simulink model "myTMSI_AnnaSparapani"  (R2017b)
settings: Solver=FixedStepAuto  StartTime=0.0  StopTime=Inf  FixedStep=0.01  RelTol=1e-3
StopFcn:
  | [file,path] = uiputfile;
  | cd(path)
  | save(file, 'EMGdata', 'EMGcount', 'QuatAngle', 'Angles', 'Angles23', 'QuatAngle1')
  | cd ..
libraries: dspindex x8
settings Model: SimulationMode=external  ExtModeTrigDuration=50000  Creator=constantin  LastModifiedBy=root
settings DataIOCC: SaveFormat=Array
settings OptimizationCC: ExpressionDepthLimit=2147483647  LifeSpan=1
settings DebuggingCC: UnderspecifiedInitializationDetection=Classic  MergeDetectMultiDrivingBlocksExec=none  SolverPrmCheckMsg=warning  StateNameClashWarn=warning  SFUnexpectedBacktrackingDiag=warning  SFNoUnconditionalDefaultTransitionDiag=warning  SFExecutionAtInitializationDiag=none
settings HardwareCC: ProdBitPerPointer=32  ProdBitPerSizeT=32  ProdBitPerPtrDiffT=32  ProdLargestAtomicFloat=None  ProdIntDivRoundTo=Undefined  ProdEndianess=Unspecified  ProdWordSize=32  ProdHWDeviceType=32-bit Generic
settings ModelReferenceCC: PropagateSignalLabelsOutOfModel=off
settings SFSimCC: MATLABDynamicMemAlloc=off
settings RTWCC: SystemTargetFile=ert_linux.tlc  MakeCommand=make_rtw OPTS=-DWITH_HW OPTIMIZATION_FLAGS=-O3  TemplateMakefile=ert_linux.tmf  Description=Linux Embedded Coder  TargetLang=C++
settings CodeAppCC: IgnoreCustomStorageClasses=off  CustomSymbolStrType=$N$R$M  StateflowObjectComments=on  InternalIdentifier=Classic
settings STFCustomTargetCC: ModelReferenceCompliant=off  CombineOutputUpdateFcns=on  ERTCustomFileBanners=on  SupportComplex=off  RemoveResetFunc=on  SupportVariableSizeSignals=on  MATLABClassNameForMDSCustomization=Simulink.SoftwareTarget.ERTCustomization  GRTInterface=off  SystemTargetFile=ert_linux.tlc
settings ERTTargetCC: MultiwordLength=2048  ModelReferenceCompliant=off  ParMdlRefBuildCompliant=off  CompOptLevelCompliant=off  ConcurrentExecutionCompliant=off  SupportComplex=off  SupportContinuousTime=on  SupportNonInlinedSFcns=on  SupportVariableSizeSignals=on  ModelStepFunctionPrototypeControlCompliant=off  CPPClassGenCompliant=off  UseToolchainInfoCompliant=off  ExtMode=on  ExtModeMexArgs='127.0.0.1' 1 17725  MultiInstanceErrorCode=None  ERTCustomFileTemplate=ert_linux_file_process.tlc  ConvertIfToSwitch=off  SuppressUnreachableDefaultCases=off
settings ConfigComp: CovMetricSettings=dw  CovHtmlReporting=on  CovSaveCumulativeToWorkspaceVar=on  CovSaveSingleToWorkspaceVar=on  CovExternalEMLEnable=off  CovSFcnEnable=off
settings SimscapeCC: SimscapeNormalizeSystem=off
settings ConfigurationSet: Description=SimMechanics 2G

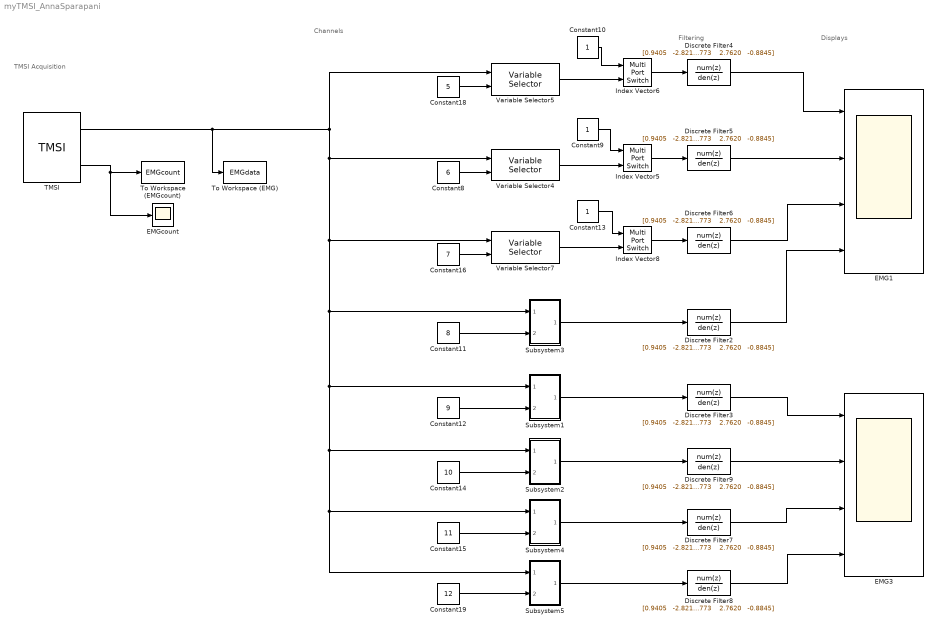
== system myTMSI_AnnaSparapani ==
  note: Displays
  note: Filtering
  note: Channels
  note: TMSI Acquisition
  Constant10 : Constant
  Constant11 : Constant  Value=8
  Constant12 : Constant  Value=9
  Constant13 : Constant
  Constant14 : Constant  Value=10
  Constant15 : Constant  Value=11
  Constant16 : Constant  Value=7
  Constant18 : Constant  Value=5
  Constant19 : Constant  Value=12
  Constant8 : Constant  Value=6
  Constant9 : Constant
  Discrete Filter{2..9} (8 alike) : DiscreteFilter  Numerator="[0.9405   -2.8214    2.8214   -0.9405]"  Denominator="[1.0000   -2.8773    2.7620   -0.8845]"
  EMG1 : Scope  NumInputPorts=4
  EMG3 : Scope  NumInputPorts=4
  EMGcount : Scope
  Index Vector5 : MultiPortSwitch  DataPortOrder=Zero-based contiguous  Inputs=1  zeroidx=on
  Index Vector6 : MultiPortSwitch  DataPortOrder=Zero-based contiguous  Inputs=1  zeroidx=on
  Index Vector8 : MultiPortSwitch  DataPortOrder=Zero-based contiguous  Inputs=1  zeroidx=on
  Subsystem1 : Subsystem
  Subsystem2 : Subsystem
  Subsystem3 : Subsystem
  Subsystem4 : Subsystem
  Subsystem5 : Subsystem
  TMSI : S-Function  FunctionName=TMSI  Parameters=uint16(frequency) int32(aux) int32(digital) int32(vectorsize) int32(ch)  SFunctionDeploymentMode=off  EnableBusSupport=off  mask{frequency=1, ch=[1 2 3 4 17 18 19 20 21 22 23 24], vectorsize=20, aux=29, digital=30}
      mask prompts: frequency "Please select a frequency"; ch "Please enter an array for channels e.g [17 29]"; vectorsize "Please enter the vector output size"; aux "Please enter the aux channel"; digital "Please enter digital channel"
      mask DialogControl DescTextVar Prompt: TMSI Block for EMG measurement
      mask Display:
      | disp('TMSI')
      | port_label('output', 1, 'data')
      | port_label('output', 2, 'status')
  To Workspace (EMG) : ToWorkspace  VariableName=EMGdata  SaveFormat=Structure With Time  SampleTime=-1
  To Workspace (EMGcount) : ToWorkspace  VariableName=EMGcount  SaveFormat=Structure With Time  SampleTime=-1
  Variable Selector4 : dspindex/Variable Selector  NumInputs=1  rowsOrCols=Rows  IdxMode=Variable  Elements=[1 3]  ZerOneIdxMode=One-based  errmode=Clip Index  FillMode=on  FillValues=0
  Variable Selector5 : dspindex/Variable Selector  NumInputs=1  rowsOrCols=Rows  IdxMode=Variable  Elements=[1 3]  ZerOneIdxMode=One-based  errmode=Clip Index  FillMode=on  FillValues=0
  Variable Selector7 : dspindex/Variable Selector  NumInputs=1  rowsOrCols=Rows  IdxMode=Variable  Elements=[1 3]  ZerOneIdxMode=One-based  errmode=Clip Index  FillMode=on  FillValues=0
  wires:
  TMSI/2 -> To Workspace (EMGcount)/1, EMGcount/1
  Index Vector6/1 -> Discrete Filter4/1
  Variable Selector4/1 -> Index Vector5/2
  Constant9/1 -> Index Vector5/1
  Variable Selector5/1 -> Index Vector6/2
  Constant10/1 -> Index Vector6/1
  Constant8/1 -> Variable Selector4/2
  Constant18/1 -> Variable Selector5/2
  Index Vector5/1 -> Discrete Filter5/1
  Index Vector8/1 -> Discrete Filter6/1
  Variable Selector7/1 -> Index Vector8/2
  Constant13/1 -> Index Vector8/1
  Constant16/1 -> Variable Selector7/2
  TMSI/1 -> Variable Selector5/1, Subsystem3/1(In1), Subsystem1/1(In1), Subsystem2/1(In1), Subsystem4/1(In1), Subsystem5/1(In1), Variable Selector7/1, Variable Selector4/1, To Workspace (EMG)/1
  Discrete Filter4/1 -> EMG1/1
  Discrete Filter5/1 -> EMG1/2
  Discrete Filter6/1 -> EMG1/3
  Constant11/1 -> Subsystem3/2(In2)
  Subsystem3/1(Out1) -> Discrete Filter2/1
  Constant12/1 -> Subsystem1/2(In2)
  Constant14/1 -> Subsystem2/2(In2)
  Constant19/1 -> Subsystem5/2(In2)
  Constant15/1 -> Subsystem4/2(In2)
  Discrete Filter2/1 -> EMG1/4
  Subsystem1/1(Out1) -> Discrete Filter3/1
  Discrete Filter3/1 -> EMG3/1
  Subsystem2/1(Out1) -> Discrete Filter9/1
  Subsystem4/1(Out1) -> Discrete Filter7/1
  Subsystem5/1(Out1) -> Discrete Filter8/1
  Discrete Filter9/1 -> EMG3/2
  Discrete Filter7/1 -> EMG3/3
  Discrete Filter8/1 -> EMG3/4

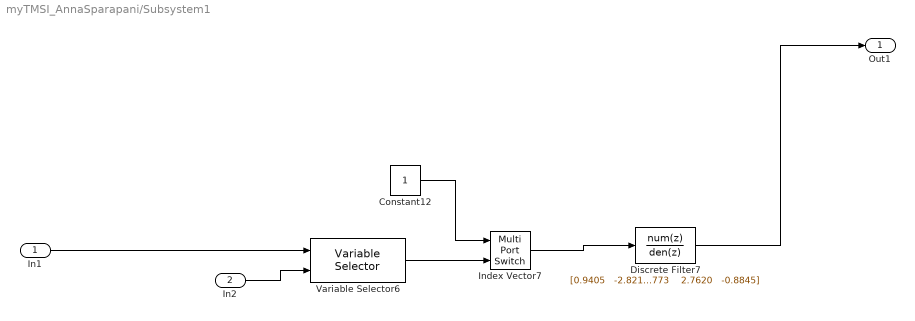
== system myTMSI_AnnaSparapani/Subsystem1 ==
  In1 : Inport
  In2 : Inport  Port=2
  Constant12 : Constant
  Discrete Filter7 : DiscreteFilter  Numerator="[0.9405   -2.8214    2.8214   -0.9405]"  Denominator="[1.0000   -2.8773    2.7620   -0.8845]"
  Index Vector7 : MultiPortSwitch  DataPortOrder=Zero-based contiguous  Inputs=1  zeroidx=on
  Variable Selector6 : dspindex/Variable Selector  NumInputs=1  rowsOrCols=Rows  IdxMode=Variable  Elements=[1 3]  ZerOneIdxMode=One-based  errmode=Clip Index  FillMode=on  FillValues=0
  Out1 : Outport
  wires:
  In1/1 -> Variable Selector6/1
  Discrete Filter7/1 -> Out1/1
  Variable Selector6/1 -> Index Vector7/2
  Constant12/1 -> Index Vector7/1
  In2/1 -> Variable Selector6/2
  Index Vector7/1 -> Discrete Filter7/1

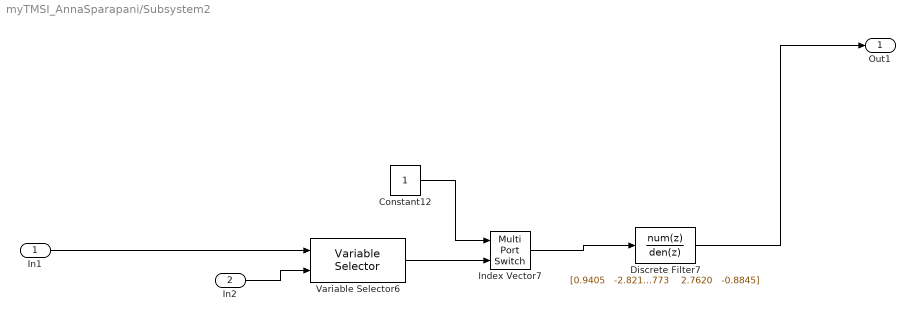
== system myTMSI_AnnaSparapani/Subsystem2 ==
  In1 : Inport
  In2 : Inport  Port=2
  Constant12 : Constant
  Discrete Filter7 : DiscreteFilter  Numerator="[0.9405   -2.8214    2.8214   -0.9405]"  Denominator="[1.0000   -2.8773    2.7620   -0.8845]"
  Index Vector7 : MultiPortSwitch  DataPortOrder=Zero-based contiguous  Inputs=1  zeroidx=on
  Variable Selector6 : dspindex/Variable Selector  NumInputs=1  rowsOrCols=Rows  IdxMode=Variable  Elements=[1 3]  ZerOneIdxMode=One-based  errmode=Clip Index  FillMode=on  FillValues=0
  Out1 : Outport
  wires:
  In1/1 -> Variable Selector6/1
  Discrete Filter7/1 -> Out1/1
  Variable Selector6/1 -> Index Vector7/2
  Constant12/1 -> Index Vector7/1
  In2/1 -> Variable Selector6/2
  Index Vector7/1 -> Discrete Filter7/1

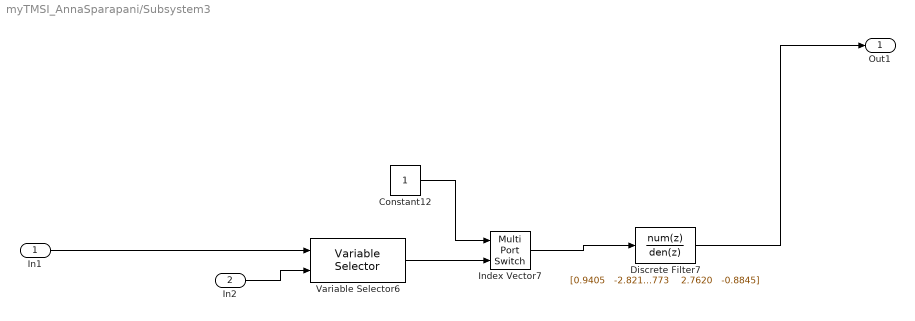
== system myTMSI_AnnaSparapani/Subsystem3 ==
  In1 : Inport
  In2 : Inport  Port=2
  Constant12 : Constant
  Discrete Filter7 : DiscreteFilter  Numerator="[0.9405   -2.8214    2.8214   -0.9405]"  Denominator="[1.0000   -2.8773    2.7620   -0.8845]"
  Index Vector7 : MultiPortSwitch  DataPortOrder=Zero-based contiguous  Inputs=1  zeroidx=on
  Variable Selector6 : dspindex/Variable Selector  NumInputs=1  rowsOrCols=Rows  IdxMode=Variable  Elements=[1 3]  ZerOneIdxMode=One-based  errmode=Clip Index  FillMode=on  FillValues=0
  Out1 : Outport
  wires:
  In1/1 -> Variable Selector6/1
  Discrete Filter7/1 -> Out1/1
  Variable Selector6/1 -> Index Vector7/2
  Constant12/1 -> Index Vector7/1
  In2/1 -> Variable Selector6/2
  Index Vector7/1 -> Discrete Filter7/1

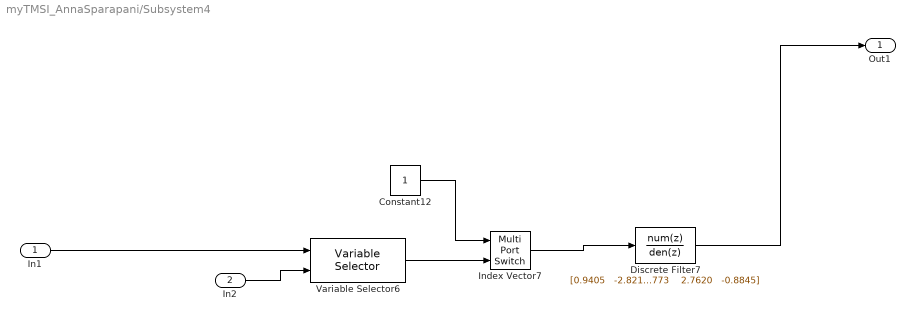
== system myTMSI_AnnaSparapani/Subsystem4 ==
  In1 : Inport
  In2 : Inport  Port=2
  Constant12 : Constant
  Discrete Filter7 : DiscreteFilter  Numerator="[0.9405   -2.8214    2.8214   -0.9405]"  Denominator="[1.0000   -2.8773    2.7620   -0.8845]"
  Index Vector7 : MultiPortSwitch  DataPortOrder=Zero-based contiguous  Inputs=1  zeroidx=on
  Variable Selector6 : dspindex/Variable Selector  NumInputs=1  rowsOrCols=Rows  IdxMode=Variable  Elements=[1 3]  ZerOneIdxMode=One-based  errmode=Clip Index  FillMode=on  FillValues=0
  Out1 : Outport
  wires:
  In1/1 -> Variable Selector6/1
  Discrete Filter7/1 -> Out1/1
  Variable Selector6/1 -> Index Vector7/2
  Constant12/1 -> Index Vector7/1
  In2/1 -> Variable Selector6/2
  Index Vector7/1 -> Discrete Filter7/1

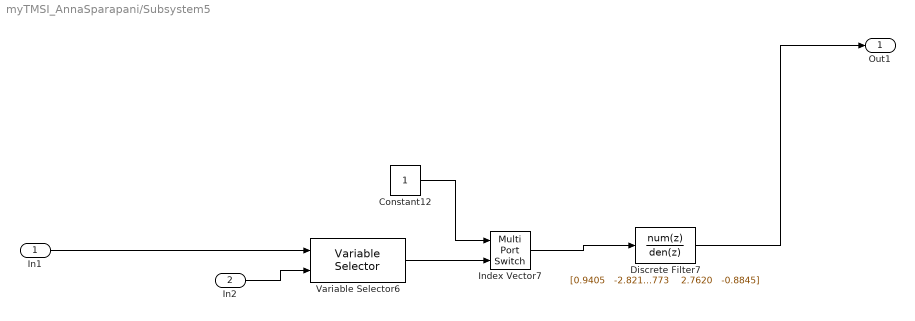
== system myTMSI_AnnaSparapani/Subsystem5 ==
  In1 : Inport
  In2 : Inport  Port=2
  Constant12 : Constant
  Discrete Filter7 : DiscreteFilter  Numerator="[0.9405   -2.8214    2.8214   -0.9405]"  Denominator="[1.0000   -2.8773    2.7620   -0.8845]"
  Index Vector7 : MultiPortSwitch  DataPortOrder=Zero-based contiguous  Inputs=1  zeroidx=on
  Variable Selector6 : dspindex/Variable Selector  NumInputs=1  rowsOrCols=Rows  IdxMode=Variable  Elements=[1 3]  ZerOneIdxMode=One-based  errmode=Clip Index  FillMode=on  FillValues=0
  Out1 : Outport
  wires:
  In1/1 -> Variable Selector6/1
  Discrete Filter7/1 -> Out1/1
  Variable Selector6/1 -> Index Vector7/2
  Constant12/1 -> Index Vector7/1
  In2/1 -> Variable Selector6/2
  Index Vector7/1 -> Discrete Filter7/1
